simulink model "hw4_4model"  (R2013a)
settings: Solver=ode45  StartTime=0.0  StopTime=t_stop  RelTol=1e-5
values from neighbouring files (symbols this model uses):
  g = 9.81    [hw4_4.m]
  k = rho*S*CD/2    (= 0.0003809)    [hw4_4.m]
  L = 0.1    [hw4_4.m]
  m = 0.01    [hw4_4.m]
  theta0 = theta_trim + delta_theta0    (= 3.19395253109)    [hw4_4.m]
  theta_dot0 = 0    [hw4_4.m]
  w = 20    [hw4_4.m]
settings Model: Creator=Willdog  LastModifiedBy=Willdog

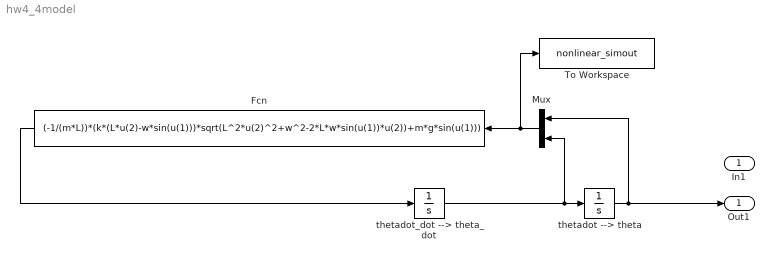
== system hw4_4model ==
  In1 : Inport
  Fcn : Fcn  Expr=(-1/(m*L))*(k*(L*u(2)-w*sin(u(1)))*sqrt(L^2*u(2)^2+w^2-2*L*w*sin(u(1))*u(2))+m*g*sin(u(1)))
  Mux : Mux  Inputs=2
  To Workspace : ToWorkspace  VariableName=nonlinear_simout  SampleTime=-1  SaveFormat=Timeseries
  thetadot --> theta : Integrator  InitialCondition=theta0
  thetadot_dot --> theta_dot : Integrator  InitialCondition=theta_dot0
  Out1 : Outport
  wires:
  thetadot --> theta/1 -> Out1/1, Mux/1
  Mux/1 -> To Workspace/1, Fcn/1
  Fcn/1 -> thetadot_dot --> theta_dot/1
  thetadot_dot --> theta_dot/1 -> Mux/2, thetadot --> theta/1
